simulink model "power_demo"  (Simulink 6.0)
settings: Solver=ode23tb  SolverMode=SingleTasking  StartTime=0.0  StopTime=.1  RelTol=1e-3
PreLoadFcn:
  | load power_demo
undefined symbols (not defined in the file or in its folder): Ki, Kp
libraries: powerlib x17, srolib x1, powerlib_extras x1
settings Model: Creator=sybille  LastModifiedBy=rlandy  ExtModeTrigMode=oneshot  ExtModeArmWhenConnect=off  ExtModeAutoUpdateStatusClock=off
settings SolverCC: MaxOrder=1
settings DataIOCC: LimitDataPoints=off  SaveOutput=off  SaveTime=off  SignalLoggingName=sigsOut
settings OptimizationCC: BlockReduction=off  BooleanDataType=off
settings DebuggingCC: CheckExecutionContextPreStartOutputMsg=on  CheckExecutionContextRuntimeOutputMsg=on  SolverPrmCheckMsg=none  UnconnectedInputMsg=none  UnconnectedOutputMsg=none
settings HardwareCC: TargetUnknown=on
settings ModelReferenceCC: UpdateModelReferenceTargets=IfOutOfDate
settings RTWCC: TemplateMakefile=grt_unix.tmf
settings SFSimCC: SFSimApplyToAllLibs=on  SFSimBuildMode=Incremental

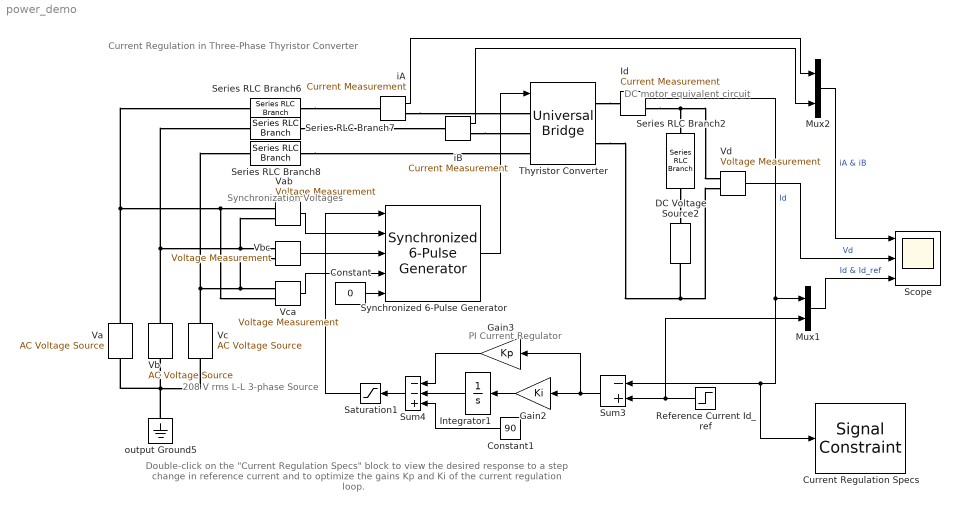
== system power_demo ==
  note: Synchronization Voltages
  note: DC motor equivalent circuit
  note: PI Current Regulator
  note: 208 V rms L-L
      | 3-phase Source
  note: Current Regulation in
      | Three-Phase Thyristor Converter
  note: Double-click on the "Current Regulation Specs" block to view
      | the desired response to a step change in reference current
      | and to optimize the gains Kp and Ki of the current regulation loop.
  Constant : Constant  Value=0
  Constant1 : Constant  Orientation=left  Value=90
  Current Regulation Specs : srolib/Signal Constraint  DialogPosition=[0.01125 0.231666666666667 0.42 0.2475]  SaveIn=workspace  SaveAs=power_optim  LogID=SRO_DataLog_1
  DC Voltage Source2 : powerlib/Electrical Sources/DC Voltage Source  Description=source block  Orientation=up  Amplitude=120  Measurements=None
      settings: AttributesFormatString=\n
  Gain2 : Gain  Orientation=left  Gain=Ki  SaturateOnIntegerOverflow=on
  Gain3 : Gain  Orientation=left  Gain=Kp  SaturateOnIntegerOverflow=on
  Id : powerlib/Measurements/Current Measurement  Tag=PoWeRsYsTeMmEaSuReMeNt  PhasorSimulation=off  OutputType=Complex  PSBequivalent=0
  Integrator1 : Integrator  Orientation=left  InitialCondition=20  LimitOutput=on  UpperSaturationLimit=160  LowerSaturationLimit=20
  Mux1 : Mux  Inputs=2
  Mux2 : Mux  Inputs=2
  Reference Current Id_ref : Step  Orientation=left  Time=0.04  Before=10  After=25  SampleTime=0
  Saturation1 : Saturate  Orientation=left  UpperLimit=160  LowerLimit=20
  Scope : Scope  NumInputPorts=3
      settings: TimeRange=0.1  YMin=-50~-200~-3.20216e-017  YMax=50~400~40  SaveName=psbconverter_str  SampleInput=on  SampleTime=1/60/512
  Series RLC Branch2 : powerlib/Elements/Series RLC Branch  Orientation=down  PhysicalDomain=powersysdomain  SubClassName=unknown  LeftPortType=p1  RightPortType=p1  LConnTagsString=__new0  RConnTagsString=__new0  Resistance=1  Inductance=20e-3  Capacitance=inf  Measurements=None
  Series RLC Branch6 : powerlib/Elements/Series RLC Branch  PhysicalDomain=powersysdomain  SubClassName=unknown  LeftPortType=p1  RightPortType=p1  LConnTagsString=__new0  RConnTagsString=__new0  Resistance=0.01  Inductance=1e-3  Capacitance=inf  Measurements=None
  Series RLC Branch7 : powerlib/Elements/Series RLC Branch  PhysicalDomain=powersysdomain  SubClassName=unknown  LeftPortType=p1  RightPortType=p1  LConnTagsString=__new0  RConnTagsString=__new0  Resistance=0.01  Inductance=1e-3  Capacitance=inf  Measurements=None
  Series RLC Branch8 : powerlib/Elements/Series RLC Branch  PhysicalDomain=powersysdomain  SubClassName=unknown  LeftPortType=p1  RightPortType=p1  LConnTagsString=__new0  RConnTagsString=__new0  Resistance=0.01  Inductance=1e-3  Capacitance=inf  Measurements=None
  Sum3 : Sum  Orientation=left  Inputs=-+  SaturateOnIntegerOverflow=on  InputSameDT=on
  Sum4 : Sum  Orientation=left  Inputs=--+  SaturateOnIntegerOverflow=on  InputSameDT=on
  Synchronized 6-Pulse Generator : powerlib_extras/Control  Blocks/Synchronized 6-Pulse Generator  freq=60  pwidth=10  Double_Pulse=on
  Thyristor Converter : powerlib/Power Electronics/Universal Bridge  Arms=3  SnubberResistance=500  SnubberCapacitance=.1e-6  Device=Thyristors  Ron=1e-3  Lon=0  ForwardVoltages="[  0.8  0.8  ]"  ForwardVoltage=.8  GTOparameters=[ 10e-6 , 20e-6 ]  IGBTparameters=[ 1e-6 , 2e-6 ]  Measurements=None
  Va : powerlib/Electrical Sources/AC Voltage Source  Description=source block  Orientation=up  Amplitude=208*sqrt(2/3)  Phase=0  Frequency=60  SampleTime=0  Measurements=None
      settings: AttributesFormatString=\n
  Vab : powerlib/Measurements/Voltage Measurement  Tag=PoWeRsYsTeMmEaSuReMeNt  PhasorSimulation=off  OutputType=Complex  PSBequivalent=0
  Vb : powerlib/Electrical Sources/AC Voltage Source  Description=source block  Orientation=up  Amplitude=208*sqrt(2/3)  Phase=-120  Frequency=60  SampleTime=0  Measurements=None
      settings: AttributesFormatString=\n
  Vbc : powerlib/Measurements/Voltage Measurement  Tag=PoWeRsYsTeMmEaSuReMeNt  PhasorSimulation=off  OutputType=Complex  PSBequivalent=0
  Vc : powerlib/Electrical Sources/AC Voltage Source  Description=source block  Orientation=up  Amplitude=208*sqrt(2/3)  Phase=120  Frequency=60  SampleTime=0  Measurements=None
      settings: AttributesFormatString=\n
  Vca : powerlib/Measurements/Voltage Measurement  Tag=PoWeRsYsTeMmEaSuReMeNt  PhasorSimulation=off  OutputType=Complex  PSBequivalent=0
  Vd : powerlib/Measurements/Voltage Measurement  Tag=PoWeRsYsTeMmEaSuReMeNt  PhasorSimulation=off  OutputType=Complex  PSBequivalent=0
  iA : powerlib/Measurements/Current Measurement  Tag=PoWeRsYsTeMmEaSuReMeNt  PhasorSimulation=off  OutputType=Complex  PSBequivalent=0
  iB : powerlib/Measurements/Current Measurement  Tag=PoWeRsYsTeMmEaSuReMeNt  PhasorSimulation=off  OutputType=Complex  PSBequivalent=0
  output Ground5 : powerlib/Elements/Ground  Orientation=down  PhysicalDomain=powersysdomain  SubClassName=unknown  LeftPortType=p1  RightPortType=p1  LConnTagsString=a
  wires:
  Gain3/1 -> Sum4/1
  Constant1/1 -> Sum4/3
  Gain2/1 -> Integrator1/1
  Sum3/1 -> Gain3/1, Gain2/1
  Sum4/1 -> Saturation1/1
  Integrator1/1 -> Sum4/2
  Saturation1/1 -> Synchronized 6-Pulse Generator/1
  Reference Current Id_ref/1 -> Sum3/2, Mux1/2
  Mux2/1 -> Scope/1  "iA & iB"
  Mux1/1 -> Scope/3  "Id & Id_ref"
  Constant/1 -> Synchronized 6-Pulse Generator/5
  Id/1 -> Mux1/1, Sum3/1, Current Regulation Specs/1  "Id"
  Vca/1 -> Synchronized 6-Pulse Generator/4
  Vbc/1 -> Synchronized 6-Pulse Generator/3
  Vab/1 -> Synchronized 6-Pulse Generator/2
  iA/1 -> Mux2/1
  iB/1 -> Mux2/2
  Vd/1 -> Scope/2  "Vd"
  Synchronized 6-Pulse Generator/1 -> Thyristor Converter/1
  connections:
  Thyristor Converter/RConn1 -- Id/LConn1
  output Ground5/LConn1 -- Vb/LConn1 -- Va/LConn1 -- Vc/LConn1
  Id/RConn1 -- Series RLC Branch2/LConn1 -- Vd/LConn1
  Series RLC Branch2/RConn1 -- DC Voltage Source2/RConn1
  Vb/RConn1 -- Vbc/LConn1 -- Vab/LConn2 -- Series RLC Branch7/LConn1
  Vc/RConn1 -- Vca/LConn1 -- Vbc/LConn2 -- Series RLC Branch8/LConn1
  Va/RConn1 -- Vab/LConn1 -- Vca/LConn2 -- Series RLC Branch6/LConn1
  Series RLC Branch8/RConn1 -- Thyristor Converter/LConn3
  Series RLC Branch6/RConn1 -- iA/LConn1
  iA/RConn1 -- Thyristor Converter/LConn1
  Series RLC Branch7/RConn1 -- iB/LConn1
  iB/RConn1 -- Thyristor Converter/LConn2
  Thyristor Converter/RConn2 -- DC Voltage Source2/LConn1 -- Vd/LConn2
